simulink model "RollCalculator"  (R2016b)
settings: Solver=VariableStepAuto  StartTime=0.0  StopTime=50  RelTol=1e-3
undefined symbols (not defined in the file): DiscIntNeverNeededParam
libraries: simulink_extras x2
settings Model: Creator=vibek  LastModifiedBy=vibek

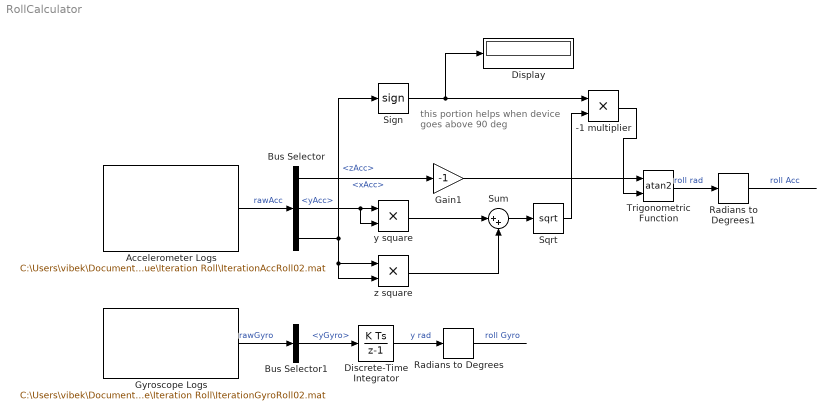
== system RollCalculator ==
  note: this portion helps when device
      | goes above 90 deg
  -1 multiplier : Product
  Accelerometer Logs : FromFile  FileName=C:\Users\vibek\Documents\MATLAB\Simulink\05.30.Tue\Iteration Roll\IterationAccRoll02.mat  OutDataTypeStr=Bus: resultAcc01  SampleTime=0.01
  Bus Selector : BusSelector  OutputSignals=xAcc,yAcc,zAcc
  Bus Selector1 : BusSelector  OutputSignals=yGyro
  Discrete-Time Integrator : DiscreteIntegrator  gainval=1  InitialConditionSetting=State (most efficient)  SampleTime=-1  ICPrevOutput=DiscIntNeverNeededParam  ICPrevScaledInput=DiscIntNeverNeededParam
  Display : Display
  Gain1 : Gain  Gain=-1
  Gyroscope Logs : FromFile  FileName=C:\Users\vibek\Documents\MATLAB\Simulink\05.30.Tue\Iteration Roll\IterationGyroRoll02.mat  OutDataTypeStr=Bus: resultGyro01  SampleTime=0.01
  Radians to Degrees : simulink_extras/Transformations/Radians to Degrees
  Radians to Degrees1 : simulink_extras/Transformations/Radians to Degrees
  Sign : Signum
  Sqrt : Sqrt  SaturateOnIntegerOverflow=on
  Sum : Sum  Inputs=|++
  Trigonometric Function : Trigonometry  Operator=atan2
  y square : Product
  "z square " : Product
  wires:
  Accelerometer Logs/1 -> Bus Selector/1  "rawAcc"
  Gyroscope Logs/1 -> Bus Selector1/1  "rawGyro"
  Bus Selector1/1 -> Discrete-Time Integrator/1  "<yGyro>"
  Discrete-Time Integrator/1 -> Radians to Degrees/1  "y rad"
  Radians to Degrees/1 -> ?  "roll Gyro"
  Bus Selector/3 -> Sign/1, "z square "/2, "z square "/1  "<zAcc>"
  "z square "/1 -> Sum/2
  Sum/1 -> Sqrt/1
  Trigonometric Function/1 -> Radians to Degrees1/1  "roll rad"
  Radians to Degrees1/1 -> ?  "roll Acc"
  Sign/1 -> Display/1, -1 multiplier/1
  Sqrt/1 -> -1 multiplier/2
  -1 multiplier/1 -> Trigonometric Function/2
  y square/1 -> Sum/1
  Bus Selector/2 -> y square/2, y square/1  "<yAcc>"
  Bus Selector/1 -> Gain1/1  "<xAcc>"
  Gain1/1 -> Trigonometric Function/1
